simulink library "LM_LIB"  (R2019b)
settings: Solver=VariableStepAuto  StartTime=0.0  StopTime=10.0  RelTol=1e-3
undefined symbols (not defined in the file): P_LM_FusBLParFiltP, P_LM_FusParC0Index, P_LM_FusParC1Index, P_LM_FusParC2Index, P_LM_FusParC3Index, P_LM_OTLBufTPMinPntNum, P_LM_OTLBufTPSPosMinDis, P_LM_OTLRearMaxDis, P_LM_OTLTPNum
libraries: simulink x84, $bdroot x3
(part 3 of 5)

== system LM_LIB/LM_LineInfo1/LM_Line_Fnt/LM_Path05 ==
  LM_FusFntPath1Dis : Inport
  LM_FusFntPath2Dis : Inport  Port=2
  LM_FusBLFntPath2C0 : Inport  Port=3
  LM_FusBLFntPath2C1 : Inport  Port=4
  LM_FusBLFntPath2C2 : Inport  Port=5
  LM_FusBLFntPath2C3 : Inport  Port=6
  LM_FusBLFntPath2Quality : Inport  Port=7
  LM_LineC0 : Inport  Port=8
  LM_FusFntPath2fCamValid : Inport  Port=9
  Add : Sum
  Bus Creator : BusCreator  Inputs=8  OutDataTypeStr=Bus: LM_TRAJINFO_BUS  NonVirtualBus=on
  Compare To Zero : simulink/Logic and Bit Operations/Compare To Zero  relop===  OutDataTypeStr=boolean
  Constant2 : Constant  Value=0  OutDataTypeStr=single
  Signal Conversion{,1..7} (8 alike) : SignalConversion  OverrideOpt=off
  Switch{,1..3} (4 alike) : Switch  Criteria=u2 ~= 0
  LM_Line05 : Outport
  wires:
  Add/1 -> Switch3/3
  LM_FusBLFntPath2C0/1 -> Add/1
  Switch3/1 -> Signal Conversion/1
  Constant2/1 -> Switch2/1, Switch1/1, Switch/1, Switch3/1
  Switch2/1 -> Signal Conversion4/1
  Switch1/1 -> Signal Conversion5/1
  LM_FusBLFntPath2Quality/1 -> Compare To Zero/1, Switch/3
  Compare To Zero/1 -> Switch/2, Switch1/2, Switch2/2, Switch3/2
  LM_FusFntPath2Dis/1 -> Switch1/3
  Signal Conversion7/1 -> Bus Creator/8  "fCamValid"
  Signal Conversion3/1 -> Bus Creator/4  "pC3"
  Bus Creator/1 -> LM_Line05/1  "LM_Line05"
  Signal Conversion2/1 -> Bus Creator/3  "pC2"
  LM_FusFntPath2fCamValid/1 -> Signal Conversion7/1
  Signal Conversion6/1 -> Bus Creator/7  "dQuality"
  LM_LineC0/1 -> Add/2
  LM_FusBLFntPath2C2/1 -> Signal Conversion2/1
  Signal Conversion5/1 -> Bus Creator/6  "dDisEnd"
  LM_FusBLFntPath2C1/1 -> Signal Conversion1/1
  Signal Conversion4/1 -> Bus Creator/5  "dDisStart"
  Switch/1 -> Signal Conversion6/1
  Signal Conversion/1 -> Bus Creator/1  "pC0"
  LM_FusBLFntPath2C3/1 -> Signal Conversion3/1
  Signal Conversion1/1 -> Bus Creator/2  "pC1"
  LM_FusFntPath1Dis/1 -> Switch2/3

== system LM_LIB/LM_LineInfo1/LM_Line_Fnt/LM_Path06 ==
  LM_LineC0 : Inport
  LM_FusBLFntPath3C0 : Inport  Port=2
  LM_FusBLFntPath3C1 : Inport  Port=3
  LM_FusBLFntPath3C2 : Inport  Port=4
  LM_FusBLFntPath3C3 : Inport  Port=5
  LM_FusBLFntPath3Quality : Inport  Port=6
  LM_FusBLFntPath2Dis : Inport  Port=7
  LM_FusBLFntPath3Dis : Inport  Port=8
  LM_FusFntPath3fCamValid : Inport  Port=9
  Add : Sum
  Bus Creator : BusCreator  Inputs=8  OutDataTypeStr=Bus: LM_TRAJINFO_BUS  NonVirtualBus=on
  Compare To Zero : simulink/Logic and Bit Operations/Compare To Zero  relop===  OutDataTypeStr=boolean
  Constant2 : Constant  Value=0  OutDataTypeStr=single
  Signal Conversion{,1..7} (8 alike) : SignalConversion  OverrideOpt=off
  Switch{,1..3} (4 alike) : Switch  Criteria=u2 ~= 0
  LM_Line06 : Outport
  wires:
  Add/1 -> Switch3/3
  LM_FusBLFntPath3C0/1 -> Add/1
  LM_FusBLFntPath3Dis/1 -> Switch1/3
  Signal Conversion5/1 -> Bus Creator/6  "dDisEnd"
  Signal Conversion3/1 -> Bus Creator/4  "pC3"
  Signal Conversion2/1 -> Bus Creator/3  "pC2"
  LM_FusBLFntPath3C1/1 -> Signal Conversion1/1
  Switch2/1 -> Signal Conversion4/1
  Signal Conversion6/1 -> Bus Creator/7  "dQuality"
  Signal Conversion7/1 -> Bus Creator/8  "fCamValid"
  LM_FusBLFntPath3C3/1 -> Signal Conversion3/1
  LM_FusFntPath3fCamValid/1 -> Signal Conversion7/1
  Signal Conversion/1 -> Bus Creator/1  "pC0"
  Signal Conversion1/1 -> Bus Creator/2  "pC1"
  LM_FusBLFntPath3C2/1 -> Signal Conversion2/1
  LM_FusBLFntPath3Quality/1 -> Compare To Zero/1, Switch/3
  Signal Conversion4/1 -> Bus Creator/5  "dDisStart"
  LM_LineC0/1 -> Add/2
  Switch3/1 -> Signal Conversion/1
  Switch1/1 -> Signal Conversion5/1
  Compare To Zero/1 -> Switch/2, Switch1/2, Switch2/2, Switch3/2
  LM_FusBLFntPath2Dis/1 -> Switch2/3
  Switch/1 -> Signal Conversion6/1
  Constant2/1 -> Switch2/1, Switch1/1, Switch/1, Switch3/1
  Bus Creator/1 -> LM_Line06/1  "LM_Line06"

== system LM_LIB/LM_LineInfo1/LM_Line_Fnt/LM_Path07 ==
  Bus Creator : BusCreator  Inputs=8  OutDataTypeStr=Bus: LM_TRAJINFO_BUS  NonVirtualBus=on
  Constant1 : Constant  Value=0  OutDataTypeStr=uint8
  Constant{2..8} (7 alike) : Constant  Value=0  OutDataTypeStr=single
  Signal Conversion{,1..7} (8 alike) : SignalConversion  OverrideOpt=off
  LM_Line07 : Outport
  wires:
  Signal Conversion5/1 -> Bus Creator/6  "dDisEnd"
  Signal Conversion3/1 -> Bus Creator/4  "pC3"
  Signal Conversion2/1 -> Bus Creator/3  "pC2"
  Signal Conversion1/1 -> Bus Creator/2  "pC1"
  Bus Creator/1 -> LM_Line07/1  "LM_Line07"
  Signal Conversion/1 -> Bus Creator/1  "pC0"
  Signal Conversion7/1 -> Bus Creator/8  "fCamValid"
  Signal Conversion6/1 -> Bus Creator/7  "dQuality"
  Signal Conversion4/1 -> Bus Creator/5  "dDisStart"
  Constant2/1 -> Signal Conversion/1
  Constant3/1 -> Signal Conversion1/1
  Constant4/1 -> Signal Conversion2/1
  Constant5/1 -> Signal Conversion3/1
  Constant6/1 -> Signal Conversion4/1
  Constant7/1 -> Signal Conversion5/1
  Constant8/1 -> Signal Conversion6/1
  Constant1/1 -> Signal Conversion7/1

== system LM_LIB/LM_LineInfo1/LM_Line_Fnt/LM_Path08 ==
  Bus Creator : BusCreator  Inputs=8  OutDataTypeStr=Bus: LM_TRAJINFO_BUS  NonVirtualBus=on
  Constant1 : Constant  Value=0  OutDataTypeStr=uint8
  Constant{2..8} (7 alike) : Constant  Value=0  OutDataTypeStr=single
  Signal Conversion{,1..7} (8 alike) : SignalConversion  OverrideOpt=off
  LM_Line08 : Outport
  wires:
  Constant8/1 -> Signal Conversion6/1
  Constant4/1 -> Signal Conversion2/1
  Constant1/1 -> Signal Conversion7/1
  Constant6/1 -> Signal Conversion4/1
  Constant3/1 -> Signal Conversion1/1
  Constant2/1 -> Signal Conversion/1
  Constant5/1 -> Signal Conversion3/1
  Signal Conversion4/1 -> Bus Creator/5  "dDisStart"
  Signal Conversion7/1 -> Bus Creator/8  "fCamValid"
  Signal Conversion1/1 -> Bus Creator/2  "pC1"
  Signal Conversion/1 -> Bus Creator/1  "pC0"
  Bus Creator/1 -> LM_Line08/1  "LM_Line08"
  Signal Conversion2/1 -> Bus Creator/3  "pC2"
  Signal Conversion3/1 -> Bus Creator/4  "pC3"
  Constant7/1 -> Signal Conversion5/1
  Signal Conversion6/1 -> Bus Creator/7  "dQuality"
  Signal Conversion5/1 -> Bus Creator/6  "dDisEnd"

== system LM_LIB/LM_LineInfo1/LM_Line_Rear/LM_Path01 ==
  LM_FusBLRearPath3C0 : Inport
  LM_FusBLRearPath3C1 : Inport  Port=2
  LM_FusBLRearPath3C2 : Inport  Port=3
  LM_FusBLRearPath3C3 : Inport  Port=4
  LM_FusBLRearPath3Quality : Inport  Port=5
  LM_LineC0 : Inport  Port=6
  LM_RearPath12Dis : Inport  Port=7
  LM_RearPath3Dis : Inport  Port=8
  Add : Sum
  Bus Creator : BusCreator  Inputs=8  OutDataTypeStr=Bus: LM_TRAJINFO_BUS  NonVirtualBus=on
  Compare To Zero : simulink/Logic and Bit Operations/Compare To Zero  relop===  OutDataTypeStr=boolean
  Constant1 : Constant  OutDataTypeStr=uint8
  Constant3 : Constant  Value=0  OutDataTypeStr=single
  Signal Conversion{,1..7} (8 alike) : SignalConversion  OverrideOpt=off
  Switch{,1..3} (4 alike) : Switch  Criteria=u2 ~= 0
  LM_Line01 : Outport
  wires:
  LM_FusBLRearPath3C0/1 -> Add/2
  Signal Conversion5/1 -> Bus Creator/6  "dDisEnd"
  Signal Conversion/1 -> Bus Creator/1  "pC0"
  Compare To Zero/1 -> Switch/2, Switch2/2, Switch3/2, Switch1/2
  Signal Conversion1/1 -> Bus Creator/2  "pC1"
  Signal Conversion2/1 -> Bus Creator/3  "pC2"
  Switch/1 -> Signal Conversion6/1
  Signal Conversion3/1 -> Bus Creator/4  "pC3"
  Switch1/1 -> Signal Conversion4/1
  Switch2/1 -> Signal Conversion5/1
  Constant3/1 -> Switch1/1, Switch2/1, Switch/1, Switch3/1
  LM_FusBLRearPath3C2/1 -> Signal Conversion2/1
  Signal Conversion4/1 -> Bus Creator/5  "dDisStart"
  Signal Conversion7/1 -> Bus Creator/8  "fCamValid"
  LM_RearPath12Dis/1 -> Switch2/3
  Add/1 -> Switch3/3
  LM_FusBLRearPath3C1/1 -> Signal Conversion1/1
  Constant1/1 -> Signal Conversion7/1
  LM_FusBLRearPath3Quality/1 -> Switch/3, Compare To Zero/1
  LM_FusBLRearPath3C3/1 -> Signal Conversion3/1
  Switch3/1 -> Signal Conversion/1
  LM_LineC0/1 -> Add/1
  Bus Creator/1 -> LM_Line01/1  "LM_Line01"
  Signal Conversion6/1 -> Bus Creator/7  "dQuality"
  LM_RearPath3Dis/1 -> Switch1/3

== system LM_LIB/LM_LineInfo1/LM_Line_Rear/LM_Path02 ==
  LM_FusBLRearPath2C0 : Inport
  LM_FusBLRearPath2C1 : Inport  Port=2
  LM_FusBLRearPath2C2 : Inport  Port=3
  LM_FusBLRearPath2C3 : Inport  Port=4
  LM_FusBLRearPath2Quality : Inport  Port=5
  LM_LineC0 : Inport  Port=6
  LM_RearPath1Dis : Inport  Port=7
  LM_RearPath2Dis : Inport  Port=8
  Add : Sum
  Bus Creator : BusCreator  Inputs=8  OutDataTypeStr=Bus: LM_TRAJINFO_BUS  NonVirtualBus=on
  Compare To Zero : simulink/Logic and Bit Operations/Compare To Zero  relop===  OutDataTypeStr=boolean
  Constant1 : Constant  OutDataTypeStr=uint8
  Constant3 : Constant  Value=0  OutDataTypeStr=single
  Signal Conversion{,1..7} (8 alike) : SignalConversion  OverrideOpt=off
  Switch{,1..3} (4 alike) : Switch  Criteria=u2 ~= 0
  LM_Line02 : Outport
  wires:
  LM_RearPath2Dis/1 -> Switch1/3
  Signal Conversion6/1 -> Bus Creator/7  "dQuality"
  Bus Creator/1 -> LM_Line02/1  "LM_Line02"
  LM_LineC0/1 -> Add/1
  Switch3/1 -> Signal Conversion/1
  LM_FusBLRearPath2C3/1 -> Signal Conversion3/1
  LM_FusBLRearPath2Quality/1 -> Compare To Zero/1, Switch/3
  Constant1/1 -> Signal Conversion7/1
  LM_FusBLRearPath2C1/1 -> Signal Conversion1/1
  Add/1 -> Switch3/3
  LM_RearPath1Dis/1 -> Switch2/3
  Signal Conversion7/1 -> Bus Creator/8  "fCamValid"
  Signal Conversion4/1 -> Bus Creator/5  "dDisStart"
  LM_FusBLRearPath2C2/1 -> Signal Conversion2/1
  Constant3/1 -> Switch3/1, Switch/1, Switch2/1, Switch1/1
  Switch2/1 -> Signal Conversion5/1
  Switch1/1 -> Signal Conversion4/1
  Signal Conversion3/1 -> Bus Creator/4  "pC3"
  Switch/1 -> Signal Conversion6/1
  Signal Conversion2/1 -> Bus Creator/3  "pC2"
  Signal Conversion1/1 -> Bus Creator/2  "pC1"
  Compare To Zero/1 -> Switch1/2, Switch3/2, Switch2/2, Switch/2
  Signal Conversion/1 -> Bus Creator/1  "pC0"
  Signal Conversion5/1 -> Bus Creator/6  "dDisEnd"
  LM_FusBLRearPath2C0/1 -> Add/2

== system LM_LIB/LM_LineInfo1/LM_Line_Rear/LM_Path03 ==
  LM_FusBLRearPath1C0 : Inport
  LM_FusBLRearPath1C1 : Inport  Port=2
  LM_FusBLRearPath1C2 : Inport  Port=3
  LM_FusBLRearPath1C3 : Inport  Port=4
  LM_FusBLRearPath1Quality : Inport  Port=5
  LM_LineC0 : Inport  Port=6
  LM_RearPath1Dis : Inport  Port=7
  Add : Sum
  Bus Creator : BusCreator  Inputs=8  OutDataTypeStr=Bus: LM_TRAJINFO_BUS  NonVirtualBus=on
  Compare To Zero : simulink/Logic and Bit Operations/Compare To Zero  relop===  OutDataTypeStr=boolean
  Constant1 : Constant  OutDataTypeStr=uint8
  Constant2 : Constant  OutDataTypeStr=single
  Constant3 : Constant  Value=0  OutDataTypeStr=single
  Constant4 : Constant  Value=0  OutDataTypeStr=single
  Product : Product
  Signal Conversion{,1..7} (8 alike) : SignalConversion  OverrideOpt=off
  Switch : Switch  Criteria=u2 ~= 0
  Switch1 : Switch  Criteria=u2 ~= 0
  Switch3 : Switch  Criteria=u2 ~= 0
  LM_Line03 : Outport
  wires:
  LM_FusBLRearPath1C0/1 -> Add/2
  Switch1/1 -> Product/1
  Signal Conversion5/1 -> Bus Creator/6  "dDisEnd"
  Signal Conversion/1 -> Bus Creator/1  "pC0"
  Compare To Zero/1 -> Switch/2, Switch3/2, Switch1/2
  Signal Conversion1/1 -> Bus Creator/2  "pC1"
  Signal Conversion2/1 -> Bus Creator/3  "pC2"
  Switch/1 -> Signal Conversion6/1
  Signal Conversion3/1 -> Bus Creator/4  "pC3"
  Product/1 -> Signal Conversion4/1
  Constant4/1 -> Signal Conversion5/1
  Constant3/1 -> Switch1/1, Switch/1, Switch3/1
  LM_FusBLRearPath1C2/1 -> Signal Conversion2/1
  Signal Conversion4/1 -> Bus Creator/5  "dDisStart"
  Signal Conversion7/1 -> Bus Creator/8  "fCamValid"
  LM_RearPath1Dis/1 -> Switch1/3
  Add/1 -> Switch3/3
  LM_FusBLRearPath1C1/1 -> Signal Conversion1/1
  Constant1/1 -> Signal Conversion7/1
  LM_FusBLRearPath1Quality/1 -> Switch/3, Compare To Zero/1
  LM_FusBLRearPath1C3/1 -> Signal Conversion3/1
  Constant2/1 -> Product/2
  Switch3/1 -> Signal Conversion/1
  LM_LineC0/1 -> Add/1
  Bus Creator/1 -> LM_Line03/1  "LM_Line03"
  Signal Conversion6/1 -> Bus Creator/7  "dQuality"

== system LM_LIB/LM_OTLBuf1InfoNew/LM_OTL_BufLe1InfoUpdate/If Action Subsystem ==
  LM_OTLBufL1Objdx : Inport
  LM_OTLBufL1Objdy : Inport  Port=2
  LM_OTLBufL1EPPos : Inport  Port=3
  LM_OTLBufL1DxVectK1Adju : Inport  Port=4
  LM_OTLBufL1DyVectK1Adju : Inport  Port=5
  Action Port : ActionPort
  Assignment : Assignment  DiagnosticForDimensions=Warning  IndexOptions=Index vector (port)  Indices=1  OutputSizes=1
  Assignment1 : Assignment  DiagnosticForDimensions=Warning  IndexOptions=Index vector (port)  Indices=1  OutputSizes=1
  Saturation : Saturate  UpperLimit=80  LowerLimit=1
  LM_OTLBufL1DxVect : Outport
  LM_OTLBufL1DyVect : Outport  Port=2
  wires:
  Assignment1/1 -> LM_OTLBufL1DyVect/1  "LM_OTLBufL1DyVect"
  Assignment/1 -> LM_OTLBufL1DxVect/1  "LM_OTLBufL1DxVect"
  LM_OTLBufL1Objdy/1 -> Assignment1/2
  LM_OTLBufL1DyVectK1Adju/1 -> Assignment1/1
  LM_OTLBufL1EPPos/1 -> Saturation/1
  LM_OTLBufL1Objdx/1 -> Assignment/2
  LM_OTLBufL1DxVectK1Adju/1 -> Assignment/1
  Saturation/1 -> Assignment/3, Assignment1/3

== system LM_LIB/LM_OTLBuf1InfoNew/LM_OTL_BufLe1InfoUpdate/If Action Subsystem1 ==
  LM_OTLBufL1DxVectK1Adju : Inport
  LM_OTLBufL1DyVectK1Adju : Inport  Port=2
  Action Port : ActionPort
  Signal Conversion : SignalConversion  OverrideOpt=off
  Signal Conversion1 : SignalConversion  OverrideOpt=off
  LM_OTLBufL1DxVect : Outport
  LM_OTLBufL1DyVect : Outport  Port=2
  wires:
  Signal Conversion1/1 -> LM_OTLBufL1DyVect/1  "LM_OTLBufL1DyVect"
  Signal Conversion/1 -> LM_OTLBufL1DxVect/1  "LM_OTLBufL1DxVect"
  LM_OTLBufL1DyVectK1Adju/1 -> Signal Conversion1/1
  LM_OTLBufL1DxVectK1Adju/1 -> Signal Conversion/1

== system LM_LIB/LM_OTLBuf1InfoNew/LM_OTL_BufLe1StoreInfoCalc/LM_OTL_ObjSICCurLeObj1InBufLe1 ==
  LM_OTLCurLeLaObj1RcdFlg : Inport
  LM_OTLCurLeLaObj1ID : Inport  Port=2
  LM_OTLCurLeLaObj1Dx : Inport  Port=3
  LM_OTLCurLeLaObj1Dy : Inport  Port=4
  LM_OTLBufL1PNumK1 : Inport  Port=5
  LM_OTLBufL1SPPosK1 : Inport  Port=6
  LM_OTLBufL1EPPosK1 : Inport  Port=7
  LM_OTLBufDxVectK1Adju : Inport  Port=8
  LM_OTLCurEgoLaObj1DyVar : Inport  Port=9
  LM_OTLCurEgoLaObj1Vy : Inport  Port=10
  LM_OTLCurEgoLaObj1VyVar : Inport  Port=11
  LM_OTLBufEgo1DyFiltHistK : Inport  Port=12
  LM_OTLBufEgo1DyVarHistK : Inport  Port=13
  psiDt : Inport  Port=14
  tDt : Inport  Port=15
  Action Port : ActionPort
  LM_OTL_BufL1DxInfo : Subsystem
  LM_OTL_BufL1DyInfo : Subsystem
  LM_OTL_BufL1EPInfo : Subsystem
  LM_OTL_BufL1IDInfo : Subsystem
  LM_OTL_BufL1PNumAndSPInfo : Subsystem
  LM_OTL_BufL1UpdateFlg : Subsystem
  LM_OTLBufL1UpdateFlg : Outport
  LM_OTLBufL1ObjID : Outport  Port=2
  LM_OTLBufL1Objdx : Outport  Port=3
  LM_OTLBufL1Objdy : Outport  Port=4
  LM_OTLBufL1ObjTPNum : Outport  Port=5
  LM_OTLBufL1ObjTPSP : Outport  Port=6
  LM_OTLBufL1ObjTPEP : Outport  Port=7
  LM_OTLBufEgo1DyVarHist : Outport  Port=8
  wires:
  LM_OTL_BufL1EPInfo/1(LM_OTLBufL1EPPos) -> LM_OTLBufL1ObjTPEP/1, [LM_OTLBufL1EPPos]
  LM_OTL_BufL1IDInfo/1(LM_OTLBufL1ObjID) -> LM_OTLBufL1ObjID/1
  LM_OTL_BufL1DxInfo/1(LM_OTLBufL1Objdx) -> LM_OTLBufL1Objdx/1
  LM_OTL_BufL1DyInfo/1(LM_OTLBufL1ObjDy) -> LM_OTLBufL1Objdy/1
  LM_OTL_BufL1PNumAndSPInfo/1(LM_OTLBufL1PNum) -> [LM_OTLBufL1ObjTPNum], LM_OTLBufL1ObjTPNum/1
  LM_OTL_BufL1PNumAndSPInfo/2(LM_OTLBufL1SPPos) -> LM_OTLBufL1ObjTPSP/1
  LM_OTL_BufL1UpdateFlg/1(LM_OTLBufL1UpdateFlg) -> LM_OTLBufL1UpdateFlg/1
  LM_OTLCurLeLaObj1RcdFlg/1 -> LM_OTL_BufL1EPInfo/1(LM_OTLCurLeLaObj1RcdFlg), LM_OTL_BufL1PNumAndSPInfo/2(LM_OTLCurLeLaObj1RcdFlg), LM_OTL_BufL1DyInfo/2(LM_OTLCurLeLaObj1RcdFlg), LM_OTL_BufL1DxInfo/2(LM_OTLCurLeLaObj1RcdFlg), LM_OTL_BufL1UpdateFlg/1(LM_OTLCurLeLaObj1RcdFlg)
  LM_OTLCurLeLaObj1ID/1 -> LM_OTL_BufL1IDInfo/1(LM_OTLCurLeLaObj1ID)
  LM_OTLCurLeLaObj1Dx/1 -> LM_OTL_BufL1DyInfo/3(LM_OTLCurLeLaObj1Dx), LM_OTL_BufL1DxInfo/1(LM_OTLCurLeLaObj1Dx)
  LM_OTLCurLeLaObj1Dy/1 -> LM_OTL_BufL1DyInfo/1(LM_OTLCurLeLaObj1Dy)
  LM_OTLBufL1PNumK1/1 -> LM_OTL_BufL1PNumAndSPInfo/1(LM_OTLBufL1PNumK1)
  LM_OTLBufL1SPPosK1/1 -> LM_OTL_BufL1PNumAndSPInfo/3(LM_OTLBufL1SPPosK1)
  LM_OTLBufL1EPPosK1/1 -> LM_OTL_BufL1EPInfo/2(LM_OTLBufL1EPPosK1)
  LM_OTLBufDxVectK1Adju/1 -> LM_OTL_BufL1PNumAndSPInfo/5(LM_OTLBufDxVectK1Adju)
  [LM_OTLBufL1EPPos] -> LM_OTL_BufL1PNumAndSPInfo/4(LM_OTLBufL1EPPos)
  LM_OTLCurEgoLaObj1DyVar/1 -> LM_OTL_BufL1DyInfo/4(LM_OTLCurEgoLaObj1DyVar)
  LM_OTLCurEgoLaObj1Vy/1 -> LM_OTL_BufL1DyInfo/5(LM_OTLCurEgoLaObj1Vy)
  LM_OTLCurEgoLaObj1VyVar/1 -> LM_OTL_BufL1DyInfo/6(LM_OTLCurEgoLaObj1VyVar)
  LM_OTLBufEgo1DyFiltHistK/1 -> LM_OTL_BufL1DyInfo/7(LM_OTLBufEgo1DyFiltHistK)
  LM_OTLBufEgo1DyVarHistK/1 -> LM_OTL_BufL1DyInfo/8(LM_OTLBufEgo1DyVarHistK)
  LM_OTL_BufL1DyInfo/2(LM_OTLBufEgo1DyVarHist) -> LM_OTLBufEgo1DyVarHist/1
  psiDt/1 -> LM_OTL_BufL1DyInfo/9(psiDt)
  tDt/1 -> LM_OTL_BufL1DyInfo/10(tDt)

== system LM_LIB/LM_OTLBuf1InfoNew/LM_OTL_BufLe1StoreInfoCalc/LM_OTL_ObjSICCurLeObj2InBufLe1 ==
  LM_OTLCurLeLaObj2RcdFlg : Inport
  LM_OTLCurLeLaObj2ID : Inport  Port=2
  LM_OTLCurLeLaObj2Dx : Inport  Port=3
  LM_OTLCurLeLaObj2Dy : Inport  Port=4
  LM_OTLBufL1PNumK1 : Inport  Port=5
  LM_OTLBufL1SPPosK1 : Inport  Port=6
  LM_OTLBufL1EPPosK1 : Inport  Port=7
  LM_OTLBufDxVectK1Adju : Inport  Port=8
  LM_OTLCurEgoLaObj2DyVar : Inport  Port=9
  LM_OTLCurEgoLaObj2Vy : Inport  Port=10
  LM_OTLCurEgoLaObj2VyVar : Inport  Port=11
  LM_OTLBufEgo2DyFiltHistK : Inport  Port=12
  LM_OTLBufEgo2DyVarHistK : Inport  Port=13
  psiDt : Inport  Port=14
  tDt : Inport  Port=15
  Action Port : ActionPort
  LM_OTL_BufL1DxInfo : Subsystem
  LM_OTL_BufL1DyInfo : Subsystem
  LM_OTL_BufL1EPInfo : Subsystem
  LM_OTL_BufL1IDInfo : Subsystem
  LM_OTL_BufL1PNumAndSPInfo : Subsystem
  LM_OTL_BufL1UpdateFlg : Subsystem
  LM_OTLBufL1UpdateFlg : Outport
  LM_OTLBufL1ObjID : Outport  Port=2
  LM_OTLBufL1Objdx : Outport  Port=3
  LM_OTLBufL1Objdy : Outport  Port=4
  LM_OTLBufL1ObjTPNum : Outport  Port=5
  LM_OTLBufL1ObjTPSP : Outport  Port=6
  LM_OTLBufL1ObjTPEP : Outport  Port=7
  LM_OTLBufEgo1DyVarHist : Outport  Port=8
  wires:
  LM_OTLBufL1PNumK1/1 -> LM_OTL_BufL1PNumAndSPInfo/1(LM_OTLBufL1PNumK1)
  LM_OTLCurLeLaObj2Dx/1 -> LM_OTL_BufL1DyInfo/1(LM_OTLCurEgoLaObj2Dx), LM_OTL_BufL1DxInfo/1(LM_OTLCurLeLaObj1Dx)
  LM_OTL_BufL1IDInfo/1(LM_OTLBufL1ObjID) -> LM_OTLBufL1ObjID/1
  [LM_OTLBufL1EPPos] -> LM_OTL_BufL1PNumAndSPInfo/4(LM_OTLBufL1EPPos)
  LM_OTL_BufL1PNumAndSPInfo/1(LM_OTLBufL1PNum) -> [LM_OTLBufL1ObjTPNum], LM_OTLBufL1ObjTPNum/1
  LM_OTLCurLeLaObj2Dy/1 -> LM_OTL_BufL1DyInfo/2(LM_OTLCurLeLaObj1Dy)
  LM_OTL_BufL1DxInfo/1(LM_OTLBufL1Objdx) -> LM_OTLBufL1Objdx/1
  LM_OTLCurLeLaObj2RcdFlg/1 -> LM_OTL_BufL1PNumAndSPInfo/2(LM_OTLCurLeLaObj2RcdFlg), LM_OTL_BufL1EPInfo/1(LM_OTLCurLeLaObj1RcdFlg), LM_OTL_BufL1DyInfo/3(LM_OTLCurLeLaObj1RcdFlg), LM_OTL_BufL1DxInfo/2(LM_OTLCurLeLaObj1RcdFlg), LM_OTL_BufL1UpdateFlg/1(LM_OTLCurLeLaObj1RcdFlg)
  LM_OTL_BufL1PNumAndSPInfo/2(LM_OTLBufL1SPPos) -> LM_OTLBufL1ObjTPSP/1
  LM_OTLCurLeLaObj2ID/1 -> LM_OTL_BufL1IDInfo/1(LM_OTLCurLeLaObj1ID)
  LM_OTL_BufL1DyInfo/1(LM_OTLBufL1ObjDy) -> LM_OTLBufL1Objdy/1
  LM_OTL_BufL1EPInfo/1(LM_OTLBufL1EPPos) -> LM_OTLBufL1ObjTPEP/1, [LM_OTLBufL1EPPos]
  LM_OTLBufL1EPPosK1/1 -> LM_OTL_BufL1EPInfo/2(LM_OTLBufL1EPPosK1)
  LM_OTL_BufL1UpdateFlg/1(LM_OTLBufL1UpdateFlg) -> LM_OTLBufL1UpdateFlg/1
  LM_OTLBufL1SPPosK1/1 -> LM_OTL_BufL1PNumAndSPInfo/3(LM_OTLBufL1SPPosK1)
  LM_OTLBufDxVectK1Adju/1 -> LM_OTL_BufL1PNumAndSPInfo/5(LM_OTLBufDxVectK1Adju)
  LM_OTLCurEgoLaObj2DyVar/1 -> LM_OTL_BufL1DyInfo/4(LM_OTLCurEgoLaObj2DyVar)
  LM_OTLCurEgoLaObj2Vy/1 -> LM_OTL_BufL1DyInfo/5(LM_OTLCurEgoLaObj2Vy)
  LM_OTLCurEgoLaObj2VyVar/1 -> LM_OTL_BufL1DyInfo/6(LM_OTLCurEgoLaObj2VyVar)
  LM_OTLBufEgo2DyFiltHistK/1 -> LM_OTL_BufL1DyInfo/7(LM_OTLBufEgo1DyFiltHistK)
  LM_OTLBufEgo2DyVarHistK/1 -> LM_OTL_BufL1DyInfo/8(LM_OTLBufEgo1DyVarHistK)
  psiDt/1 -> LM_OTL_BufL1DyInfo/9(psiDt)
  tDt/1 -> LM_OTL_BufL1DyInfo/10(tDt)
  LM_OTL_BufL1DyInfo/2(LM_OTLBufEgo1DyVarHist) -> LM_OTLBufEgo1DyVarHist/1

== system LM_LIB/LM_OTLBuf1InfoNew/LM_OTL_BufLe1StoreInfoCalc/LM_OTL_ObjSICNoCurObjInBufLe1 ==
  LM_OTLCurLeLaObj1Index : Inport
  LM_OTLCurLeLaObj2Index : Inport  Port=2
  LM_OTLCurLeLaObj1RcdedFlg : Inport  Port=3
  LM_OTLCurLeLaObj1ID : Inport  Port=4
  LM_OTLCurLeLaObj2ID : Inport  Port=5
  LM_OTLCurLeLaObj1Dx : Inport  Port=6
  LM_OTLCurLeLaObj2Dx : Inport  Port=7
  LM_OTLCurLeLaObj1Dy : Inport  Port=8
  LM_OTLCurLeLaObj2Dy : Inport  Port=9
  LM_OTLBufL1LastTPValid : Inport  Port=10
  LM_OTLBufL1LastEPPos : Inport  Port=11
  LM_OTLCurEgoLaObj1DyVar : Inport  Port=12
  LM_OTLCurEgoLaObj2DyVar : Inport  Port=13
  Action Port : ActionPort
  LM_OTL_BufL1DxInfo : Subsystem
  LM_OTL_BufL1DyInfo : Subsystem
  LM_OTL_BufL1DyInfo1 : Subsystem
  LM_OTL_BufL1EPInfo : Subsystem
  LM_OTL_BufL1IDInfo : Subsystem
  LM_OTL_BufL1PNumInfo : Subsystem
  LM_OTL_BufL1SPInfo : Subsystem
  LM_OTLBufL1UpdateFlg : Outport
  LM_OTLBufL1ObjID : Outport  Port=2
  LM_OTLBufL1Objdx : Outport  Port=3
  LM_OTLBufL1Objdy : Outport  Port=4
  LM_OTLBufL1ObjTPNum : Outport  Port=5
  LM_OTLBufL1ObjTPSP : Outport  Port=6
  LM_OTLBufL1ObjTPEP : Outport  Port=7
  LM_OTLBufEgo1DyVarHist : Outport  Port=8
  wires:
  LM_OTL_BufL1IDInfo/2(LM_OTLBufL1ObjID) -> LM_OTLBufL1ObjID/1
  LM_OTL_BufL1DxInfo/1(LM_OTLBufL1Objdx) -> LM_OTLBufL1Objdx/1
  LM_OTL_BufL1DyInfo/1(LM_OTLBufL1Objdy) -> LM_OTLBufL1Objdy/1
  LM_OTL_BufL1PNumInfo/1(LM_OTLBufL1TPNum) -> LM_OTLBufL1ObjTPNum/1
  LM_OTL_BufL1SPInfo/1(LM_OTLBufL1SPPos) -> LM_OTL_BufL1EPInfo/1(LM_OTLBufL1SPPos), LM_OTLBufL1ObjTPSP/1
  LM_OTL_BufL1EPInfo/1(LM_OTLBufL1EPPos) -> LM_OTLBufL1ObjTPEP/1
  LM_OTLCurLeLaObj1ID/1 -> LM_OTL_BufL1IDInfo/4(LM_OTLCurLeLaObj1ID)
  LM_OTLCurLeLaObj2ID/1 -> LM_OTL_BufL1IDInfo/5(LM_OTLCurLeLaObj2ID)
  LM_OTLCurLeLaObj1Dx/1 -> LM_OTL_BufL1DxInfo/4(LM_OTLCurLeLaObj1Dx)
  LM_OTLCurLeLaObj2Dx/1 -> LM_OTL_BufL1DxInfo/5(LM_OTLCurLeLaObj2Dx)
  LM_OTLCurLeLaObj2Dy/1 -> LM_OTL_BufL1DyInfo/5(LM_OTLCurLeLaObj2Dy)
  LM_OTLCurLeLaObj1Dy/1 -> LM_OTL_BufL1DyInfo/4(LM_OTLCurLeLaObj1Dy)
  LM_OTLBufL1LastTPValid/1 -> LM_OTL_BufL1SPInfo/4(LM_OTLBufL1LastTPValid)
  LM_OTLBufL1LastEPPos/1 -> LM_OTL_BufL1SPInfo/5(LM_OTLBufL1LastEPPos)
  LM_OTL_BufL1IDInfo/1(LM_OTLBufL1UpdateFlg) -> LM_OTLBufL1UpdateFlg/1
  LM_OTLCurEgoLaObj2DyVar/1 -> LM_OTL_BufL1DyInfo1/5(LM_OTLCurEgoLaObj2DyVar)
  LM_OTLCurEgoLaObj1DyVar/1 -> LM_OTL_BufL1DyInfo1/4(LM_OTLCurEgoLaObj1DyVar)
  LM_OTLCurLeLaObj1RcdedFlg/1 -> LM_OTL_BufL1DyInfo1/3(LM_OTLCurLeLaObj1RcdedFlg), LM_OTL_BufL1SPInfo/3(LM_OTLCurLeLaObj1RcdedFlg), LM_OTL_BufL1PNumInfo/3(LM_OTLCurLeLaObj1RcdedFlg), LM_OTL_BufL1DyInfo/3(LM_OTLCurLeLaObj1RcdedFlg), LM_OTL_BufL1DxInfo/3(LM_OTLCurLeLaObj1RcdedFlg), LM_OTL_BufL1IDInfo/3(LM_OTLCurLeLaObj1RcdedFlg)
  LM_OTLCurLeLaObj2Index/1 -> LM_OTL_BufL1DyInfo1/2(LM_OTLCurLeLaObj2Index), LM_OTL_BufL1SPInfo/2(LM_OTLCurLeLaObj2Index), LM_OTL_BufL1PNumInfo/2(LM_OTLCurLeLaObj2Index), LM_OTL_BufL1DyInfo/2(LM_OTLCurLeLaObj2Index), LM_OTL_BufL1DxInfo/2(LM_OTLCurLeLaObj2Index), LM_OTL_BufL1IDInfo/2(LM_OTLCurLeLaObj2Index)
  LM_OTLCurLeLaObj1Index/1 -> LM_OTL_BufL1DyInfo1/1(LM_OTLCurLeLaObj1Index), LM_OTL_BufL1SPInfo/1(LM_OTLCurLeLaObj1Index), LM_OTL_BufL1PNumInfo/1(LM_OTLCurLeLaObj1Index), LM_OTL_BufL1DyInfo/1(LM_OTLCurLeLaObj1Index), LM_OTL_BufL1DxInfo/1(LM_OTLCurLeLaObj1Index), LM_OTL_BufL1IDInfo/1(LM_OTLCurLeLaObj1Index)
  LM_OTL_BufL1DyInfo1/1(LM_OTLBufEgo1DyVarHist) -> LM_OTLBufEgo1DyVarHist/1

== system LM_LIB/LM_OTLBuf2InfoNew/LM_OTL_BufLe1InfoUpdate/If Action Subsystem ==
  LM_OTLBufL1Objdx : Inport
  LM_OTLBufL1Objdy : Inport  Port=2
  LM_OTLBufL1EPPos : Inport  Port=3
  LM_OTLBufL1DxVectK1Adju : Inport  Port=4
  LM_OTLBufL1DyVectK1Adju : Inport  Port=5
  Action Port : ActionPort
  Assignment : Assignment  DiagnosticForDimensions=Warning  IndexOptions=Index vector (port)  Indices=1  OutputSizes=1
  Assignment1 : Assignment  DiagnosticForDimensions=Warning  IndexOptions=Index vector (port)  Indices=1  OutputSizes=1
  Saturation : Saturate  UpperLimit=80  LowerLimit=1
  LM_OTLBufL1DxVect : Outport
  LM_OTLBufL1DyVect : Outport  Port=2
  wires:
  Assignment1/1 -> LM_OTLBufL1DyVect/1  "LM_OTLBufL1DyVect"
  Assignment/1 -> LM_OTLBufL1DxVect/1  "LM_OTLBufL1DxVect"
  LM_OTLBufL1Objdy/1 -> Assignment1/2
  LM_OTLBufL1DyVectK1Adju/1 -> Assignment1/1
  LM_OTLBufL1EPPos/1 -> Saturation/1
  LM_OTLBufL1Objdx/1 -> Assignment/2
  LM_OTLBufL1DxVectK1Adju/1 -> Assignment/1
  Saturation/1 -> Assignment/3, Assignment1/3

== system LM_LIB/LM_OTLBuf2InfoNew/LM_OTL_BufLe1InfoUpdate/If Action Subsystem1 ==
  LM_OTLBufL1DxVectK1Adju : Inport
  LM_OTLBufL1DyVectK1Adju : Inport  Port=2
  Action Port : ActionPort
  Signal Conversion : SignalConversion  OverrideOpt=off
  Signal Conversion1 : SignalConversion  OverrideOpt=off
  LM_OTLBufL1DxVect : Outport
  LM_OTLBufL1DyVect : Outport  Port=2
  wires:
  Signal Conversion1/1 -> LM_OTLBufL1DyVect/1  "LM_OTLBufL1DyVect"
  Signal Conversion/1 -> LM_OTLBufL1DxVect/1  "LM_OTLBufL1DxVect"
  LM_OTLBufL1DyVectK1Adju/1 -> Signal Conversion1/1
  LM_OTLBufL1DxVectK1Adju/1 -> Signal Conversion/1

== system LM_LIB/LM_OTLBuf2InfoNew/LM_OTL_BufLe1StoreInfoCalc/LM_OTL_ObjSICCurLeObj1InBufLe1 ==
  LM_OTLCurLeLaObj1RcdFlg : Inport
  LM_OTLCurLeLaObj1ID : Inport  Port=2
  LM_OTLCurLeLaObj1Dx : Inport  Port=3
  LM_OTLCurLeLaObj1Dy : Inport  Port=4
  LM_OTLBufL1PNumK1 : Inport  Port=5
  LM_OTLBufL1SPPosK1 : Inport  Port=6
  LM_OTLBufL1EPPosK1 : Inport  Port=7
  LM_OTLBufDxVectK1Adju : Inport  Port=8
  LM_OTLCurEgoLaObj1DyVar : Inport  Port=9
  LM_OTLCurEgoLaObj1Vy : Inport  Port=10
  LM_OTLCurEgoLaObj1VyVar : Inport  Port=11
  LM_OTLBufEgo1DyFiltHistK : Inport  Port=12
  LM_OTLBufEgo1DyVarHistK : Inport  Port=13
  psiDt : Inport  Port=14
  tDt : Inport  Port=15
  Action Port : ActionPort
  LM_OTL_BufL1DxInfo : Subsystem
  LM_OTL_BufL1DyInfo : Subsystem
  LM_OTL_BufL1EPInfo : Subsystem
  LM_OTL_BufL1IDInfo : Subsystem
  LM_OTL_BufL1PNumAndSPInfo : Subsystem
  LM_OTL_BufL1UpdateFlg : Subsystem
  LM_OTLBufL1UpdateFlg : Outport
  LM_OTLBufL1ObjID : Outport  Port=2
  LM_OTLBufL1Objdx : Outport  Port=3
  LM_OTLBufL1Objdy : Outport  Port=4
  LM_OTLBufL1ObjTPNum : Outport  Port=5
  LM_OTLBufL1ObjTPSP : Outport  Port=6
  LM_OTLBufL1ObjTPEP : Outport  Port=7
  LM_OTLBufEgo1DyVarHist : Outport  Port=8
  wires:
  LM_OTL_BufL1EPInfo/1(LM_OTLBufL1EPPos) -> LM_OTLBufL1ObjTPEP/1, [LM_OTLBufL1EPPos]
  LM_OTL_BufL1IDInfo/1(LM_OTLBufL1ObjID) -> LM_OTLBufL1ObjID/1
  LM_OTL_BufL1DxInfo/1(LM_OTLBufL1Objdx) -> LM_OTLBufL1Objdx/1
  LM_OTL_BufL1DyInfo/1(LM_OTLBufL1ObjDy) -> LM_OTLBufL1Objdy/1
  LM_OTL_BufL1PNumAndSPInfo/1(LM_OTLBufL1PNum) -> [LM_OTLBufL1ObjTPNum], LM_OTLBufL1ObjTPNum/1
  LM_OTL_BufL1PNumAndSPInfo/2(LM_OTLBufL1SPPos) -> LM_OTLBufL1ObjTPSP/1
  LM_OTL_BufL1UpdateFlg/1(LM_OTLBufL1UpdateFlg) -> LM_OTLBufL1UpdateFlg/1
  LM_OTLCurLeLaObj1RcdFlg/1 -> LM_OTL_BufL1EPInfo/1(LM_OTLCurLeLaObj1RcdFlg), LM_OTL_BufL1PNumAndSPInfo/2(LM_OTLCurLeLaObj1RcdFlg), LM_OTL_BufL1DyInfo/2(LM_OTLCurLeLaObj1RcdFlg), LM_OTL_BufL1DxInfo/2(LM_OTLCurLeLaObj1RcdFlg), LM_OTL_BufL1UpdateFlg/1(LM_OTLCurLeLaObj1RcdFlg)
  LM_OTLCurLeLaObj1ID/1 -> LM_OTL_BufL1IDInfo/1(LM_OTLCurLeLaObj1ID)
  LM_OTLCurLeLaObj1Dx/1 -> LM_OTL_BufL1DyInfo/3(LM_OTLCurLeLaObj1Dx), LM_OTL_BufL1DxInfo/1(LM_OTLCurLeLaObj1Dx)
  LM_OTLCurLeLaObj1Dy/1 -> LM_OTL_BufL1DyInfo/1(LM_OTLCurLeLaObj1Dy)
  LM_OTLBufL1PNumK1/1 -> LM_OTL_BufL1PNumAndSPInfo/1(LM_OTLBufL1PNumK1)
  LM_OTLBufL1SPPosK1/1 -> LM_OTL_BufL1PNumAndSPInfo/3(LM_OTLBufL1SPPosK1)
  LM_OTLBufL1EPPosK1/1 -> LM_OTL_BufL1EPInfo/2(LM_OTLBufL1EPPosK1)
  LM_OTLBufDxVectK1Adju/1 -> LM_OTL_BufL1PNumAndSPInfo/5(LM_OTLBufDxVectK1Adju)
  [LM_OTLBufL1EPPos] -> LM_OTL_BufL1PNumAndSPInfo/4(LM_OTLBufL1EPPos)
  LM_OTLCurEgoLaObj1DyVar/1 -> LM_OTL_BufL1DyInfo/4(LM_OTLCurEgoLaObj1DyVar)
  LM_OTLCurEgoLaObj1Vy/1 -> LM_OTL_BufL1DyInfo/5(LM_OTLCurEgoLaObj1Vy)
  LM_OTLCurEgoLaObj1VyVar/1 -> LM_OTL_BufL1DyInfo/6(LM_OTLCurEgoLaObj1VyVar)
  LM_OTLBufEgo1DyFiltHistK/1 -> LM_OTL_BufL1DyInfo/7(LM_OTLBufEgo1DyFiltHistK)
  LM_OTLBufEgo1DyVarHistK/1 -> LM_OTL_BufL1DyInfo/8(LM_OTLBufEgo1DyVarHistK)
  LM_OTL_BufL1DyInfo/2(LM_OTLBufEgo1DyVarHist) -> LM_OTLBufEgo1DyVarHist/1
  psiDt/1 -> LM_OTL_BufL1DyInfo/9(psiDt)
  tDt/1 -> LM_OTL_BufL1DyInfo/10(tDt)

== system LM_LIB/LM_OTLBuf2InfoNew/LM_OTL_BufLe1StoreInfoCalc/LM_OTL_ObjSICCurLeObj2InBufLe1 ==
  LM_OTLCurLeLaObj2RcdFlg : Inport
  LM_OTLCurLeLaObj2ID : Inport  Port=2
  LM_OTLCurLeLaObj2Dx : Inport  Port=3
  LM_OTLCurLeLaObj2Dy : Inport  Port=4
  LM_OTLBufL1PNumK1 : Inport  Port=5
  LM_OTLBufL1SPPosK1 : Inport  Port=6
  LM_OTLBufL1EPPosK1 : Inport  Port=7
  LM_OTLBufDxVectK1Adju : Inport  Port=8
  LM_OTLCurEgoLaObj2DyVar : Inport  Port=9
  LM_OTLCurEgoLaObj2Vy : Inport  Port=10
  LM_OTLCurEgoLaObj2VyVar : Inport  Port=11
  LM_OTLBufEgo2DyFiltHistK : Inport  Port=12
  LM_OTLBufEgo2DyVarHistK : Inport  Port=13
  psiDt : Inport  Port=14
  tDt : Inport  Port=15
  Action Port : ActionPort
  LM_OTL_BufL1DxInfo : Subsystem
  LM_OTL_BufL1DyInfo : Subsystem
  LM_OTL_BufL1EPInfo : Subsystem
  LM_OTL_BufL1IDInfo : Subsystem
  LM_OTL_BufL1PNumAndSPInfo : Subsystem
  LM_OTL_BufL1UpdateFlg : Subsystem
  LM_OTLBufL1UpdateFlg : Outport
  LM_OTLBufL1ObjID : Outport  Port=2
  LM_OTLBufL1Objdx : Outport  Port=3
  LM_OTLBufL1Objdy : Outport  Port=4
  LM_OTLBufL1ObjTPNum : Outport  Port=5
  LM_OTLBufL1ObjTPSP : Outport  Port=6
  LM_OTLBufL1ObjTPEP : Outport  Port=7
  LM_OTLBufEgo1DyVarHist : Outport  Port=8
  wires:
  LM_OTLBufL1PNumK1/1 -> LM_OTL_BufL1PNumAndSPInfo/1(LM_OTLBufL1PNumK1)
  LM_OTLCurLeLaObj2Dx/1 -> LM_OTL_BufL1DyInfo/1(LM_OTLCurEgoLaObj2Dx), LM_OTL_BufL1DxInfo/1(LM_OTLCurLeLaObj1Dx)
  LM_OTL_BufL1IDInfo/1(LM_OTLBufL1ObjID) -> LM_OTLBufL1ObjID/1
  [LM_OTLBufL1EPPos] -> LM_OTL_BufL1PNumAndSPInfo/4(LM_OTLBufL1EPPos)
  LM_OTL_BufL1PNumAndSPInfo/1(LM_OTLBufL1PNum) -> [LM_OTLBufL1ObjTPNum], LM_OTLBufL1ObjTPNum/1
  LM_OTLCurLeLaObj2Dy/1 -> LM_OTL_BufL1DyInfo/2(LM_OTLCurLeLaObj1Dy)
  LM_OTL_BufL1DxInfo/1(LM_OTLBufL1Objdx) -> LM_OTLBufL1Objdx/1
  LM_OTLCurLeLaObj2RcdFlg/1 -> LM_OTL_BufL1PNumAndSPInfo/2(LM_OTLCurLeLaObj2RcdFlg), LM_OTL_BufL1EPInfo/1(LM_OTLCurLeLaObj1RcdFlg), LM_OTL_BufL1DyInfo/3(LM_OTLCurLeLaObj1RcdFlg), LM_OTL_BufL1DxInfo/2(LM_OTLCurLeLaObj1RcdFlg), LM_OTL_BufL1UpdateFlg/1(LM_OTLCurLeLaObj1RcdFlg)
  LM_OTL_BufL1PNumAndSPInfo/2(LM_OTLBufL1SPPos) -> LM_OTLBufL1ObjTPSP/1
  LM_OTLCurLeLaObj2ID/1 -> LM_OTL_BufL1IDInfo/1(LM_OTLCurLeLaObj1ID)
  LM_OTL_BufL1DyInfo/1(LM_OTLBufL1ObjDy) -> LM_OTLBufL1Objdy/1
  LM_OTL_BufL1EPInfo/1(LM_OTLBufL1EPPos) -> LM_OTLBufL1ObjTPEP/1, [LM_OTLBufL1EPPos]
  LM_OTLBufL1EPPosK1/1 -> LM_OTL_BufL1EPInfo/2(LM_OTLBufL1EPPosK1)
  LM_OTL_BufL1UpdateFlg/1(LM_OTLBufL1UpdateFlg) -> LM_OTLBufL1UpdateFlg/1
  LM_OTLBufL1SPPosK1/1 -> LM_OTL_BufL1PNumAndSPInfo/3(LM_OTLBufL1SPPosK1)
  LM_OTLBufDxVectK1Adju/1 -> LM_OTL_BufL1PNumAndSPInfo/5(LM_OTLBufDxVectK1Adju)
  LM_OTLCurEgoLaObj2DyVar/1 -> LM_OTL_BufL1DyInfo/4(LM_OTLCurEgoLaObj2DyVar)
  LM_OTLCurEgoLaObj2Vy/1 -> LM_OTL_BufL1DyInfo/5(LM_OTLCurEgoLaObj2Vy)
  LM_OTLCurEgoLaObj2VyVar/1 -> LM_OTL_BufL1DyInfo/6(LM_OTLCurEgoLaObj2VyVar)
  LM_OTLBufEgo2DyFiltHistK/1 -> LM_OTL_BufL1DyInfo/7(LM_OTLBufEgo1DyFiltHistK)
  LM_OTLBufEgo2DyVarHistK/1 -> LM_OTL_BufL1DyInfo/8(LM_OTLBufEgo1DyVarHistK)
  psiDt/1 -> LM_OTL_BufL1DyInfo/9(psiDt)
  tDt/1 -> LM_OTL_BufL1DyInfo/10(tDt)
  LM_OTL_BufL1DyInfo/2(LM_OTLBufEgo1DyVarHist) -> LM_OTLBufEgo1DyVarHist/1

== system LM_LIB/LM_OTLBuf2InfoNew/LM_OTL_BufLe1StoreInfoCalc/LM_OTL_ObjSICNoCurObjInBufLe1 ==
  LM_OTLCurLeLaObj1Index1 : Inport
  LM_OTLCurLeLaObj2Index1 : Inport  Port=2
  LM_OTLCurLeLaObj1RcdedFlg1 : Inport  Port=3
  LM_OTLCurLeLaObj1ID1 : Inport  Port=4
  LM_OTLCurLeLaObj2ID1 : Inport  Port=5
  LM_OTLCurLeLaObj1Dx : Inport  Port=6
  LM_OTLCurLeLaObj2Dx : Inport  Port=7
  LM_OTLCurLeLaObj1Dy : Inport  Port=8
  LM_OTLCurLeLaObj2Dy : Inport  Port=9
  LM_OTLBufL1LastTPValid1 : Inport  Port=10
  LM_OTLBufL1LastEPPos1 : Inport  Port=11
  LM_OTLBuf1ID1 : Inport  Port=12
  LM_OTLCurEgoLaObj1DyVar1 : Inport  Port=13
  LM_OTLCurEgoLaObj2DyVar1 : Inport  Port=14
  Action Port : ActionPort
  LM_OTL_BufL1IDInfo1 : Subsystem
  LM_OTL_BufL1PNumInfo1 : Subsystem
  LM_OTL_BufL1SPInfo1 : Subsystem
  LM_OTL_BufL2EPInfo : Subsystem
  LM_OTL_BufL2PosInfo : Subsystem
  LM_OTLBuf2UpdateFlg : Outport
  LM_OTLBuf2ObjID : Outport  Port=2
  LM_OTLBuf2Objdx : Outport  Port=3
  LM_OTLBuf2Objdy : Outport  Port=4
  LM_OTLBuf2ObjTPNum : Outport  Port=5
  LM_OTLBuf2ObjTPSP : Outport  Port=6
  LM_OTLBuf2ObjTPEP : Outport  Port=7
  LM_OTLBuf2DyVarHist : Outport  Port=8
  wires:
  LM_OTL_BufL1IDInfo1/2(LM_OTLBuf2ObjID) -> LM_OTL_BufL1SPInfo1/1(LM_OTLBufL2ObjID), LM_OTL_BufL1PNumInfo1/1(LM_OTLBufL2ObjID), LM_OTL_BufL2PosInfo/1(LM_OTLBufL2ObjID), LM_OTLBuf2ObjID/1
  LM_OTL_BufL2PosInfo/1(LM_OTLBuf2Objdx) -> LM_OTLBuf2Objdx/1
  LM_OTL_BufL1SPInfo1/1(LM_OTLBuf2SPPos) -> LM_OTLBuf2ObjTPSP/1, LM_OTL_BufL2EPInfo/1(LM_OTLBufL2SPPos)
  LM_OTL_BufL2EPInfo/1(LM_OTLBuf2EPPos) -> LM_OTLBuf2ObjTPEP/1
  LM_OTLCurLeLaObj1Index1/1 -> LM_OTL_BufL1IDInfo1/2(LM_OTLCurLeLaObj1Index)
  LM_OTLBufL1LastTPValid1/1 -> LM_OTL_BufL1SPInfo1/2(LM_OTLBufL2LastTPValid)
  LM_OTLCurLeLaObj1ID1/1 -> LM_OTL_BufL1IDInfo1/5(LM_OTLCurLeLaObj1ID), LM_OTL_BufL2PosInfo/2(LM_OTLCurLeLaObj1ID)
  LM_OTLCurLeLaObj2Index1/1 -> LM_OTL_BufL1IDInfo1/3(LM_OTLCurLeLaObj2Index)
  LM_OTLBuf1ID1/1 -> LM_OTL_BufL1IDInfo1/1(LM_OTLBuf1ID)
  LM_OTLCurLeLaObj1RcdedFlg1/1 -> LM_OTL_BufL1IDInfo1/4(LM_OTLCurLeLaObj1RcdedFlg)
  LM_OTLCurLeLaObj2Dy/1 -> LM_OTL_BufL2PosInfo/7(LM_OTLCurLeLaObj2Dy)
  LM_OTL_BufL1IDInfo1/1(LM_OTLBuf2UpdateFlg) -> LM_OTLBuf2UpdateFlg/1
  LM_OTLCurLeLaObj1Dy/1 -> LM_OTL_BufL2PosInfo/6(LM_OTLCurLeLaObj1Dy)
  LM_OTLCurLeLaObj2ID1/1 -> LM_OTL_BufL1IDInfo1/6(LM_OTLCurLeLaObj2ID), LM_OTL_BufL2PosInfo/3(LM_OTLCurLeLaObj2ID)
  LM_OTL_BufL1PNumInfo1/1(LM_OTLBuf2TPNum) -> LM_OTLBuf2ObjTPNum/1
  LM_OTLCurLeLaObj1Dx/1 -> LM_OTL_BufL2PosInfo/4(LM_OTLCurLeLaObj1Dx)
  LM_OTLCurLeLaObj2Dx/1 -> LM_OTL_BufL2PosInfo/5(LM_OTLCurLeLaObj2Dx)
  LM_OTLBufL1LastEPPos1/1 -> LM_OTL_BufL1SPInfo1/3(LM_OTLBufL2LastEPPos)
  LM_OTL_BufL2PosInfo/2(LM_OTLBuf2Objdy) -> LM_OTLBuf2Objdy/1
  LM_OTLCurEgoLaObj1DyVar1/1 -> LM_OTL_BufL2PosInfo/8(LM_OTLCurEgoLaObj1DyVar)
  LM_OTLCurEgoLaObj2DyVar1/1 -> LM_OTL_BufL2PosInfo/9(LM_OTLCurEgoLaObj2DyVar)
  LM_OTL_BufL2PosInfo/3(LM_OTLBuf2DyVarHist) -> LM_OTLBuf2DyVarHist/1

== system LM_LIB/LM_OTLBufLostTPValidJudgeNew/If Action Subsystem/If Action Subsystem ==
  LM_OTLBufLastPNumK1 : Inport
  LM_OTLBufLastSPPosK1 : Inport  Port=2
  LM_OTLBufLastEPPosK1 : Inport  Port=3
  LM_OTLBufL1DxVectK1Adju : Inport  Port=4
  LM_OTLBufPNumK1 : Inport  Port=5
  LM_OTLBufSPPosK1 : Inport  Port=6
  LM_OTLBufEPPosK1 : Inport  Port=7
  Action Port : ActionPort  ActionPortLabel=if(u1 > 0)
  If : If  IfExpression=u1 ~= 0
  If Action Subsystem : Subsystem  TreatAsAtomicUnit=on
  If Action Subsystem1 : Subsystem  TreatAsAtomicUnit=on
  LM_OTL_Last1ObjTPValidJudge : Subsystem
  LM_OTL_Last1ObjValidTPDisClac : Subsystem
  Merge{,1..3} (4 alike) : Merge
  LM_OTLBufLastTPValid : Outport
  LM_OTLBufLastPNum : Outport  Port=2
  LM_OTLBufLastSPPos : Outport  Port=3
  LM_OTLBufLastEPPos : Outport  Port=4
  wires:
  LM_OTL_Last1ObjValidTPDisClac/1(LM_OTLLast1ObjValidTPDis) -> LM_OTL_Last1ObjTPValidJudge/1(LM_OTLLast1ObjValidTPDis)
  LM_OTL_Last1ObjTPValidJudge/1(LM_OTLLast1ObjTPValid) -> If/1
  If/1 -> If Action Subsystem/Action
  If/2 -> If Action Subsystem1/Action
  LM_OTLBufL1DxVectK1Adju/1 -> If Action Subsystem1/1(LM_OTLBufDxVectK1Adju), LM_OTL_Last1ObjValidTPDisClac/1(LM_OTLBufL1DxVectK1Adju)
  LM_OTLBufSPPosK1/1 -> If Action Subsystem/1(LM_OTLBufSPPosK1), LM_OTL_Last1ObjValidTPDisClac/2(LM_OTLBufSPPosK1)
  LM_OTLBufEPPosK1/1 -> If Action Subsystem/2(LM_OTLBufEPPosK1), LM_OTL_Last1ObjValidTPDisClac/3(LM_OTLBufEPPosK1)
  LM_OTLBufPNumK1/1 -> If Action Subsystem/3(LM_OTLBufPNumK1)
  LM_OTLBufLastSPPosK1/1 -> If Action Subsystem1/3(LM_OTLBufLastSPPosK1)
  LM_OTLBufLastPNumK1/1 -> If Action Subsystem1/2(LM_OTLBufLastPNumK1)
  LM_OTLBufLastEPPosK1/1 -> If Action Subsystem1/4(LM_OTLBufLastEPPosK1)
  If Action Subsystem/1(LM_OTLBufLastTPValid) -> Merge/1
  If Action Subsystem/2(LM_OTLBufLastPNum) -> Merge1/1
  If Action Subsystem/3(LM_OTLBufLastSPPos) -> Merge2/1
  If Action Subsystem/4(LM_OTLBufLastEPPos) -> Merge3/1
  If Action Subsystem1/1(LM_OTLBufLastTPValid) -> Merge/2
  If Action Subsystem1/2(LM_OTLBufLastPNum) -> Merge1/2
  If Action Subsystem1/3(LM_OTLBufLastSPPos) -> Merge2/2
  If Action Subsystem1/4(LM_OTLBufLastEPPos) -> Merge3/2
  Merge/1 -> LM_OTLBufLastTPValid/1  "LM_OTLBufLastTPValid"
  Merge1/1 -> LM_OTLBufLastPNum/1  "LM_OTLBufLastPNum"
  Merge2/1 -> LM_OTLBufLastSPPos/1  "LM_OTLBufLastSPPos"
  Merge3/1 -> LM_OTLBufLastEPPos/1  "LM_OTLBufLastEPPos"

== system LM_LIB/LM_OTLBufLostTPValidJudgeNew/If Action Subsystem/If Action Subsystem1 ==
  LM_OTLBufL1DxVectK1Adju : Inport
  LM_OTLBufPNumK1 : Inport  Port=2
  LM_OTLBufSPPosK1 : Inport  Port=3
  LM_OTLBufEPPosK1 : Inport  Port=4
  Action Port : ActionPort  ActionPortLabel=else
  LM_OTL_Last1ObjTPValidJudge : Subsystem
  LM_OTL_Last1ObjValidTPDisClac : Subsystem
  LM_OTL_LastObjInfoCalc : Subsystem
  LM_OTLBufLastTPValid : Outport
  LM_OTLBufLastPNum : Outport  Port=2
  LM_OTLBufLastSPPos : Outport  Port=3
  LM_OTLBufLastEPPos : Outport  Port=4
  wires:
  LM_OTLBufL1DxVectK1Adju/1 -> LM_OTL_Last1ObjValidTPDisClac/1(LM_OTLBufL1DxVectK1Adju)
  LM_OTLBufSPPosK1/1 -> LM_OTL_LastObjInfoCalc/2(LM_OTLBufSPPosK1), LM_OTL_Last1ObjValidTPDisClac/2(LM_OTLBufSPPosK1)
  LM_OTLBufEPPosK1/1 -> LM_OTL_LastObjInfoCalc/3(LM_OTLBufEPPosK1), LM_OTL_Last1ObjValidTPDisClac/3(LM_OTLBufEPPosK1)
  LM_OTL_Last1ObjValidTPDisClac/1(LM_OTLLast1ObjValidTPDis) -> LM_OTL_Last1ObjTPValidJudge/1(LM_OTLLast1ObjValidTPDis)
  LM_OTL_Last1ObjTPValidJudge/1(LM_OTLLast1ObjTPValid) -> LM_OTL_LastObjInfoCalc/1(LM_OTLLast1ObjTPValid)
  LM_OTL_LastObjInfoCalc/1(LM_OTLBufLastTPValid) -> LM_OTLBufLastTPValid/1
  LM_OTL_LastObjInfoCalc/2(LM_OTLBufLastPNum) -> LM_OTLBufLastPNum/1
  LM_OTL_LastObjInfoCalc/3(LM_OTLBufLastSPPos) -> LM_OTLBufLastSPPos/1
  LM_OTL_LastObjInfoCalc/4(LM_OTLBufLastEPPos) -> LM_OTLBufLastEPPos/1
  LM_OTLBufPNumK1/1 -> LM_OTL_LastObjInfoCalc/4(LM_OTLBufPNumK1)

== system LM_LIB/LM_OTL_Buf1InfoUpdate/LM_OTL_BufLe1InfoUpdate/If Action Subsystem ==
  LM_OTLBufL1Objdx : Inport
  LM_OTLBufL1Objdy : Inport  Port=2
  LM_OTLBufL1EPPos : Inport  Port=3
  LM_OTLBufL1DxVectK1Adju : Inport  Port=4
  LM_OTLBufL1DyVectK1Adju : Inport  Port=5
  Action Port : ActionPort
  Assignment : Assignment  DiagnosticForDimensions=Warning  IndexOptions=Index vector (port)  Indices=1  OutputSizes=1
  Assignment1 : Assignment  DiagnosticForDimensions=Warning  IndexOptions=Index vector (port)  Indices=1  OutputSizes=1
  LM_OTLBufL1DxVect : Outport
  LM_OTLBufL1DyVect : Outport  Port=2
  wires:
  Assignment1/1 -> LM_OTLBufL1DyVect/1  "LM_OTLBufL1DyVect"
  Assignment/1 -> LM_OTLBufL1DxVect/1  "LM_OTLBufL1DxVect"
  LM_OTLBufL1Objdy/1 -> Assignment1/2
  LM_OTLBufL1DyVectK1Adju/1 -> Assignment1/1
  LM_OTLBufL1EPPos/1 -> Assignment/3, Assignment1/3
  LM_OTLBufL1Objdx/1 -> Assignment/2
  LM_OTLBufL1DxVectK1Adju/1 -> Assignment/1

== system LM_LIB/LM_OTL_Buf1InfoUpdate/LM_OTL_BufLe1InfoUpdate/If Action Subsystem1 ==
  LM_OTLBufL1DxVectK1Adju : Inport
  LM_OTLBufL1DyVectK1Adju : Inport  Port=2
  Action Port : ActionPort
  Signal Conversion : SignalConversion  OverrideOpt=off
  Signal Conversion1 : SignalConversion  OverrideOpt=off
  LM_OTLBufL1DxVect : Outport
  LM_OTLBufL1DyVect : Outport  Port=2
  wires:
  Signal Conversion1/1 -> LM_OTLBufL1DyVect/1  "LM_OTLBufL1DyVect"
  Signal Conversion/1 -> LM_OTLBufL1DxVect/1  "LM_OTLBufL1DxVect"
  LM_OTLBufL1DyVectK1Adju/1 -> Signal Conversion1/1
  LM_OTLBufL1DxVectK1Adju/1 -> Signal Conversion/1

== system LM_LIB/LM_OTL_Buf1InfoUpdate/LM_OTL_BufLe1StoreInfoCalc/LM_OTL_ObjSICCurLeObj1InBufLe1 ==
  LM_OTLCurLeLaObj1RcdFlg : Inport
  LM_OTLCurLeLaObj1ID : Inport  Port=2
  LM_OTLCurLeLaObj1Dx : Inport  Port=3
  LM_OTLCurLeLaObj1Dy : Inport  Port=4
  LM_OTLBufL1PNumK1 : Inport  Port=5
  LM_OTLBufL1SPPosK1 : Inport  Port=6
  LM_OTLBufL1EPPosK1 : Inport  Port=7
  LM_OTLBufDxVectK1Adju : Inport  Port=8
  Action Port : ActionPort
  LM_OTL_BufL1DxInfo : Subsystem
  LM_OTL_BufL1DyInfo : Subsystem
  LM_OTL_BufL1EPInfo : Subsystem
  LM_OTL_BufL1IDInfo : Subsystem
  LM_OTL_BufL1PNumAndSPInfo : Subsystem
  LM_OTL_BufL1UpdateFlg : Subsystem
  LM_OTLBufL1UpdateFlg : Outport
  LM_OTLBufL1ObjID : Outport  Port=2
  LM_OTLBufL1Objdx : Outport  Port=3
  LM_OTLBufL1Objdy : Outport  Port=4
  LM_OTLBufL1ObjTPNum : Outport  Port=5
  LM_OTLBufL1ObjTPSP : Outport  Port=6
  LM_OTLBufL1ObjTPEP : Outport  Port=7
  wires:
  LM_OTL_BufL1EPInfo/1(LM_OTLBufL1EPPos) -> LM_OTLBufL1ObjTPEP/1, [LM_OTLBufL1EPPos]
  LM_OTL_BufL1IDInfo/1(LM_OTLBufL1ObjID) -> LM_OTLBufL1ObjID/1
  LM_OTL_BufL1DxInfo/1(LM_OTLBufL1Objdx) -> LM_OTLBufL1Objdx/1
  LM_OTL_BufL1DyInfo/1(LM_OTLBufL1ObjDy) -> LM_OTLBufL1Objdy/1
  LM_OTL_BufL1PNumAndSPInfo/1(LM_OTLBufL1PNum) -> [LM_OTLBufL1ObjTPNum], LM_OTLBufL1ObjTPNum/1
  LM_OTL_BufL1PNumAndSPInfo/2(LM_OTLBufL1SPPos) -> LM_OTLBufL1ObjTPSP/1
  LM_OTL_BufL1UpdateFlg/1(LM_OTLBufL1UpdateFlg) -> LM_OTLBufL1UpdateFlg/1
  LM_OTLCurLeLaObj1RcdFlg/1 -> LM_OTL_BufL1EPInfo/1(LM_OTLCurLeLaObj1RcdFlg), LM_OTL_BufL1PNumAndSPInfo/2(LM_OTLCurLeLaObj1RcdFlg), LM_OTL_BufL1DyInfo/2(LM_OTLCurLeLaObj1RcdFlg), LM_OTL_BufL1DxInfo/2(LM_OTLCurLeLaObj1RcdFlg), LM_OTL_BufL1UpdateFlg/1(LM_OTLCurLeLaObj1RcdFlg)
  LM_OTLCurLeLaObj1ID/1 -> LM_OTL_BufL1IDInfo/1(LM_OTLCurLeLaObj1ID)
  LM_OTLCurLeLaObj1Dx/1 -> LM_OTL_BufL1DxInfo/1(LM_OTLCurLeLaObj1Dx)
  LM_OTLCurLeLaObj1Dy/1 -> LM_OTL_BufL1DyInfo/1(LM_OTLCurLeLaObj1Dy)
  LM_OTLBufL1PNumK1/1 -> LM_OTL_BufL1PNumAndSPInfo/1(LM_OTLBufL1PNumK1)
  LM_OTLBufL1SPPosK1/1 -> LM_OTL_BufL1PNumAndSPInfo/3(LM_OTLBufL1SPPosK1)
  LM_OTLBufL1EPPosK1/1 -> LM_OTL_BufL1EPInfo/2(LM_OTLBufL1EPPosK1)
  LM_OTLBufDxVectK1Adju/1 -> LM_OTL_BufL1PNumAndSPInfo/5(LM_OTLBufDxVectK1Adju)
  [LM_OTLBufL1EPPos] -> LM_OTL_BufL1PNumAndSPInfo/4(LM_OTLBufL1EPPos)

== system LM_LIB/LM_OTL_Buf1InfoUpdate/LM_OTL_BufLe1StoreInfoCalc/LM_OTL_ObjSICCurLeObj2InBufLe1 ==
  LM_OTLCurLeLaObj2RcdFlg : Inport
  LM_OTLCurLeLaObj2ID : Inport  Port=2
  LM_OTLCurLeLaObj2Dx : Inport  Port=3
  LM_OTLCurLeLaObj2Dy : Inport  Port=4
  LM_OTLBufL1PNumK1 : Inport  Port=5
  LM_OTLBufL1SPPosK1 : Inport  Port=6
  LM_OTLBufL1EPPosK1 : Inport  Port=7
  LM_OTLBufDxVectK1Adju : Inport  Port=8
  Action Port : ActionPort
  LM_OTL_BufL1DxInfo : Subsystem
  LM_OTL_BufL1DyInfo : Subsystem
  LM_OTL_BufL1EPInfo : Subsystem
  LM_OTL_BufL1IDInfo : Subsystem
  LM_OTL_BufL1PNumAndSPInfo : Subsystem
  LM_OTL_BufL1UpdateFlg : Subsystem
  LM_OTLBufL1UpdateFlg : Outport
  LM_OTLBufL1ObjID : Outport  Port=2
  LM_OTLBufL1Objdx : Outport  Port=3
  LM_OTLBufL1Objdy : Outport  Port=4
  LM_OTLBufL1ObjTPNum : Outport  Port=5
  LM_OTLBufL1ObjTPSP : Outport  Port=6
  LM_OTLBufL1ObjTPEP : Outport  Port=7
  wires:
  LM_OTLBufL1PNumK1/1 -> LM_OTL_BufL1PNumAndSPInfo/1(LM_OTLBufL1PNumK1)
  LM_OTLCurLeLaObj2Dx/1 -> LM_OTL_BufL1DxInfo/1(LM_OTLCurLeLaObj1Dx)
  LM_OTL_BufL1IDInfo/1(LM_OTLBufL1ObjID) -> LM_OTLBufL1ObjID/1
  [LM_OTLBufL1EPPos] -> LM_OTL_BufL1PNumAndSPInfo/4(LM_OTLBufL1EPPos)
  LM_OTL_BufL1PNumAndSPInfo/1(LM_OTLBufL1PNum) -> [LM_OTLBufL1ObjTPNum], LM_OTLBufL1ObjTPNum/1
  LM_OTLCurLeLaObj2Dy/1 -> LM_OTL_BufL1DyInfo/1(LM_OTLCurLeLaObj1Dy)
  LM_OTL_BufL1DxInfo/1(LM_OTLBufL1Objdx) -> LM_OTLBufL1Objdx/1
  LM_OTLCurLeLaObj2RcdFlg/1 -> LM_OTL_BufL1PNumAndSPInfo/2(LM_OTLCurLeLaObj2RcdFlg), LM_OTL_BufL1EPInfo/1(LM_OTLCurLeLaObj1RcdFlg), LM_OTL_BufL1DyInfo/2(LM_OTLCurLeLaObj1RcdFlg), LM_OTL_BufL1DxInfo/2(LM_OTLCurLeLaObj1RcdFlg), LM_OTL_BufL1UpdateFlg/1(LM_OTLCurLeLaObj1RcdFlg)
  LM_OTL_BufL1PNumAndSPInfo/2(LM_OTLBufL1SPPos) -> LM_OTLBufL1ObjTPSP/1
  LM_OTLCurLeLaObj2ID/1 -> LM_OTL_BufL1IDInfo/1(LM_OTLCurLeLaObj1ID)
  LM_OTL_BufL1DyInfo/1(LM_OTLBufL1ObjDy) -> LM_OTLBufL1Objdy/1
  LM_OTL_BufL1EPInfo/1(LM_OTLBufL1EPPos) -> LM_OTLBufL1ObjTPEP/1, [LM_OTLBufL1EPPos]
  LM_OTLBufL1EPPosK1/1 -> LM_OTL_BufL1EPInfo/2(LM_OTLBufL1EPPosK1)
  LM_OTL_BufL1UpdateFlg/1(LM_OTLBufL1UpdateFlg) -> LM_OTLBufL1UpdateFlg/1
  LM_OTLBufL1SPPosK1/1 -> LM_OTL_BufL1PNumAndSPInfo/3(LM_OTLBufL1SPPosK1)
  LM_OTLBufDxVectK1Adju/1 -> LM_OTL_BufL1PNumAndSPInfo/5(LM_OTLBufDxVectK1Adju)

== system LM_LIB/LM_OTL_Buf1InfoUpdate/LM_OTL_BufLe1StoreInfoCalc/LM_OTL_ObjSICNoCurObjInBufLe1 ==
  LM_OTLCurLeLaObj1Index : Inport
  LM_OTLCurLeLaObj2Index : Inport  Port=2
  LM_OTLCurLeLaObj1RcdedFlg : Inport  Port=3
  LM_OTLCurLeLaObj1ID : Inport  Port=4
  LM_OTLCurLeLaObj2ID : Inport  Port=5
  LM_OTLCurLeLaObj1Dx : Inport  Port=6
  LM_OTLCurLeLaObj2Dx : Inport  Port=7
  LM_OTLCurLeLaObj1Dy : Inport  Port=8
  LM_OTLCurLeLaObj2Dy : Inport  Port=9
  LM_OTLBufL1LastTPValid : Inport  Port=10
  LM_OTLBufL1LastEPPos : Inport  Port=11
  Action Port : ActionPort
  LM_OTL_BufL1DxInfo : Subsystem
  LM_OTL_BufL1DyInfo : Subsystem
  LM_OTL_BufL1EPInfo : Subsystem
  LM_OTL_BufL1IDInfo : Subsystem
  LM_OTL_BufL1PNumInfo : Subsystem
  LM_OTL_BufL1SPInfo : Subsystem
  LM_OTLBufL1UpdateFlg : Outport
  LM_OTLBufL1ObjID : Outport  Port=2
  LM_OTLBufL1Objdx : Outport  Port=3
  LM_OTLBufL1Objdy : Outport  Port=4
  LM_OTLBufL1ObjTPNum : Outport  Port=5
  LM_OTLBufL1ObjTPSP : Outport  Port=6
  LM_OTLBufL1ObjTPEP : Outport  Port=7
  wires:
  LM_OTL_BufL1IDInfo/2(LM_OTLBufL1ObjID) -> LM_OTLBufL1ObjID/1
  LM_OTL_BufL1DxInfo/1(LM_OTLBufL1Objdx) -> LM_OTLBufL1Objdx/1
  LM_OTL_BufL1DyInfo/1(LM_OTLBufL1Objdy) -> LM_OTLBufL1Objdy/1
  LM_OTL_BufL1PNumInfo/1(LM_OTLBufL1TPNum) -> LM_OTLBufL1ObjTPNum/1
  LM_OTL_BufL1SPInfo/1(LM_OTLBufL1SPPos) -> LM_OTL_BufL1EPInfo/1(LM_OTLBufL1SPPos), LM_OTLBufL1ObjTPSP/1
  LM_OTL_BufL1EPInfo/1(LM_OTLBufL1EPPos) -> LM_OTLBufL1ObjTPEP/1
  LM_OTLCurLeLaObj1Index/1 -> LM_OTL_BufL1SPInfo/1(LM_OTLCurLeLaObj1Index), LM_OTL_BufL1PNumInfo/1(LM_OTLCurLeLaObj1Index), LM_OTL_BufL1DyInfo/1(LM_OTLCurLeLaObj1Index), LM_OTL_BufL1DxInfo/1(LM_OTLCurLeLaObj1Index), LM_OTL_BufL1IDInfo/1(LM_OTLCurLeLaObj1Index)
  LM_OTLCurLeLaObj2Index/1 -> LM_OTL_BufL1SPInfo/2(LM_OTLCurLeLaObj2Index), LM_OTL_BufL1PNumInfo/2(LM_OTLCurLeLaObj2Index), LM_OTL_BufL1DyInfo/2(LM_OTLCurLeLaObj2Index), LM_OTL_BufL1DxInfo/2(LM_OTLCurLeLaObj2Index), LM_OTL_BufL1IDInfo/2(LM_OTLCurLeLaObj2Index)
  LM_OTLCurLeLaObj1RcdedFlg/1 -> LM_OTL_BufL1SPInfo/3(LM_OTLCurLeLaObj1RcdedFlg), LM_OTL_BufL1PNumInfo/3(LM_OTLCurLeLaObj1RcdedFlg), LM_OTL_BufL1DyInfo/3(LM_OTLCurLeLaObj1RcdedFlg), LM_OTL_BufL1DxInfo/3(LM_OTLCurLeLaObj1RcdedFlg), LM_OTL_BufL1IDInfo/3(LM_OTLCurLeLaObj1RcdedFlg)
  LM_OTLCurLeLaObj1ID/1 -> LM_OTL_BufL1IDInfo/4(LM_OTLCurLeLaObj1ID)
  LM_OTLCurLeLaObj2ID/1 -> LM_OTL_BufL1IDInfo/5(LM_OTLCurLeLaObj2ID)
  LM_OTLCurLeLaObj1Dx/1 -> LM_OTL_BufL1DxInfo/4(LM_OTLCurLeLaObj1Dx)
  LM_OTLCurLeLaObj2Dx/1 -> LM_OTL_BufL1DxInfo/5(LM_OTLCurLeLaObj2Dx)
  LM_OTLCurLeLaObj2Dy/1 -> LM_OTL_BufL1DyInfo/5(LM_OTLCurLeLaObj2Dy)
  LM_OTLCurLeLaObj1Dy/1 -> LM_OTL_BufL1DyInfo/4(LM_OTLCurLeLaObj1Dy)
  LM_OTLBufL1LastTPValid/1 -> LM_OTL_BufL1SPInfo/4(LM_OTLBufL1LastTPValid)
  LM_OTLBufL1LastEPPos/1 -> LM_OTL_BufL1SPInfo/5(LM_OTLBufL1LastEPPos)
  LM_OTL_BufL1IDInfo/1(LM_OTLBufL1UpdateFlg) -> LM_OTLBufL1UpdateFlg/1

== system LM_LIB/LM_OTL_Buf2InfoUpdate/LM_OTL_BufLe1InfoUpdate/If Action Subsystem ==
  LM_OTLBufL1Objdx : Inport
  LM_OTLBufL1Objdy : Inport  Port=2
  LM_OTLBufL1EPPos : Inport  Port=3
  LM_OTLBufL1DxVectK1Adju : Inport  Port=4
  LM_OTLBufL1DyVectK1Adju : Inport  Port=5
  Action Port : ActionPort
  Assignment : Assignment  DiagnosticForDimensions=Warning  IndexOptions=Index vector (port)  Indices=1  OutputSizes=1
  Assignment1 : Assignment  DiagnosticForDimensions=Warning  IndexOptions=Index vector (port)  Indices=1  OutputSizes=1
  LM_OTLBufL1DxVect : Outport
  LM_OTLBufL1DyVect : Outport  Port=2
  wires:
  Assignment1/1 -> LM_OTLBufL1DyVect/1  "LM_OTLBufL1DyVect"
  Assignment/1 -> LM_OTLBufL1DxVect/1  "LM_OTLBufL1DxVect"
  LM_OTLBufL1Objdy/1 -> Assignment1/2
  LM_OTLBufL1DyVectK1Adju/1 -> Assignment1/1
  LM_OTLBufL1EPPos/1 -> Assignment/3, Assignment1/3
  LM_OTLBufL1Objdx/1 -> Assignment/2
  LM_OTLBufL1DxVectK1Adju/1 -> Assignment/1

== system LM_LIB/LM_OTL_Buf2InfoUpdate/LM_OTL_BufLe1InfoUpdate/If Action Subsystem1 ==
  LM_OTLBufL1DxVectK1Adju : Inport
  LM_OTLBufL1DyVectK1Adju : Inport  Port=2
  Action Port : ActionPort
  Signal Conversion : SignalConversion  OverrideOpt=off
  Signal Conversion1 : SignalConversion  OverrideOpt=off
  LM_OTLBufL1DxVect : Outport
  LM_OTLBufL1DyVect : Outport  Port=2
  wires:
  Signal Conversion1/1 -> LM_OTLBufL1DyVect/1  "LM_OTLBufL1DyVect"
  Signal Conversion/1 -> LM_OTLBufL1DxVect/1  "LM_OTLBufL1DxVect"
  LM_OTLBufL1DyVectK1Adju/1 -> Signal Conversion1/1
  LM_OTLBufL1DxVectK1Adju/1 -> Signal Conversion/1
